simulink model "TST_StateflowDefaultTransitionCondition"  (Simulink 10.0)
settings: Solver=FixedStepDiscrete  StartTime=0.0  StopTime=10.0  FixedStep=0.02  RelTol=1e-3  EnableMultiTasking=on
settings Model: Creator=kharthforeign  LastModifiedBy=unknown
settings DataIOCC: LimitDataPoints=on  SignalLoggingSaveFormat=ModelDataLogs  SaveOutput=off  SignalLogging=off  SaveTime=off
settings OptimizationCC: BlockReduction=off  ConditionallyExecuteInputs=off  OptimizeBlockIOStorage=off  BufferReuse=off  GlobalBufferReuse=off  ExpressionFolding=off  ExpressionDepthLimit=2147483647  LocalBlockOutputs=off  InitFltsAndDblsToZero=on  OptimizeDataStoreBuffers=off  BusAssignmentInplaceUpdate=off
settings DebuggingCC: SolverPrmCheckMsg=warning  FcnCallInpInsideContextMsg=warning  StateNameClashWarn=warning
settings SFSimCC: SimParseCustomCode=off
settings GRTTargetCC: GeneratePreprocessorConditionals=Disable all
settings ConfigComp: CovExternalEMLEnable=off

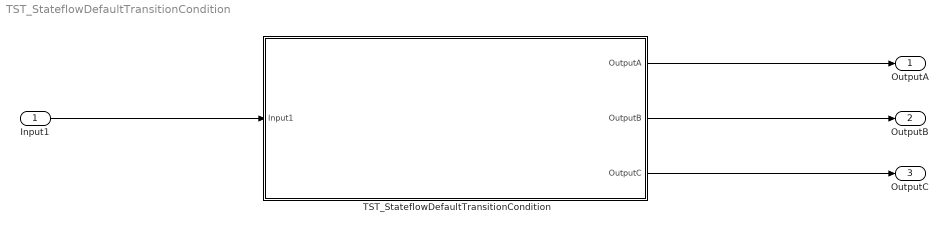
== system TST_StateflowDefaultTransitionCondition ==
  Input1 : Inport  OutDataTypeStr=uint32  BusOutputAsStruct=on
  TST_StateflowDefaultTransitionCondition : Subsystem  TreatAsAtomicUnit=on
  OutputA : Outport  OutDataTypeStr=double  PortDimensions=1
  OutputB : Outport  Port=2  OutDataTypeStr=double  PortDimensions=1
  OutputC : Outport  Port=3  OutDataTypeStr=double  PortDimensions=1
  wires:
  Input1/1 -> TST_StateflowDefaultTransitionCondition/1(Input1)
  TST_StateflowDefaultTransitionCondition/1(OutputA) -> OutputA/1
  TST_StateflowDefaultTransitionCondition/2(OutputB) -> OutputB/1
  TST_StateflowDefaultTransitionCondition/3(OutputC) -> OutputC/1

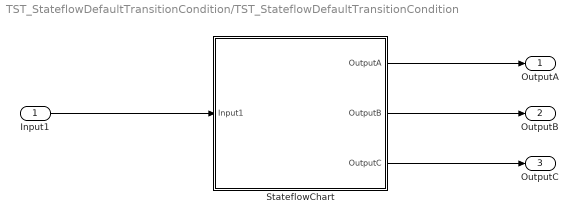
== system TST_StateflowDefaultTransitionCondition/TST_StateflowDefaultTransitionCondition ==
  Input1 : Inport  OutDataTypeStr=uint32  BusOutputAsStruct=on
  StateflowChart : Stateflow chart  TreatAsAtomicUnit=on
  OutputA : Outport  OutDataTypeStr=double  PortDimensions=1
  OutputB : Outport  Port=2  OutDataTypeStr=double  PortDimensions=1
  OutputC : Outport  Port=3  OutDataTypeStr=double  PortDimensions=1
  wires:
  StateflowChart/1(OutputA) -> OutputA/1
  StateflowChart/2(OutputB) -> OutputB/1
  StateflowChart/3(OutputC) -> OutputC/1
  Input1/1 -> StateflowChart/1(Input1)

== stateflow chart TST_StateflowDefaultTransitionCondition/StateflowChart ==
  state StateA
    entry:
    OutputA = 10.0;
  state StateB
    entry:
    OutputB = 20.0;
    state Ping
    state Pong
    (default) -> Ping
    Ping -> Pong : [A]
    Pong -> Ping : [B]
  state ResultA = EvaluateConditionA(X) [function]
    (default) -> (junction 14) : [X > 123.0]...
        | {ResultA = false;}
  state ResultB = EvaluateConditionB(X) [function]
    (default) -> (junction 19)
    (junction 19) -> (junction 18) : [X > 123.0]...
        | {ResultB = false;}
  (default) -> StateA : [A && B]...
      | {Local = 5.0;}
  StateA -> StateB : [EvaluateConditionB(Local)]
  StateB -> StateA : [EvaluateConditionA(-1.0 * Local)]
  data: X function_input double; ResultA function_output boolean =true; X function_input double; ResultB function_output boolean =true; Input1 input uint32; OutputA output double =1; OutputB output double =2; OutputC output double =3; Local local double =0; A local boolean; B local boolean; C local boolean
